simulink model "nid_cvst_ir"  (Simulink 7.6)
settings: Solver=FixedStepDiscrete  StartTime=0.0  StopTime=inf  RelTol=1e-3
libraries: vipsnks x2, nid_lib x2
settings Model: Creator=tchikama  LastModifiedBy=tchikama
settings DataIOCC: SaveOutput=off
settings OptimizationCC: SimCompilerOptimization=On
settings HardwareCC: ProdIntDivRoundTo=Zero  ProdEndianess=LittleEndian  ProdHWDeviceType=Generic->32-bit x86 compatible
settings RTWCC: ProcessScript=grt_make_rtw_hook  RTWCompilerOptimization=On
settings CodeAppCC: MaxIdLength=95

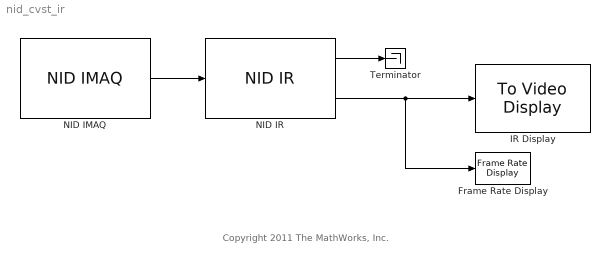
== system nid_cvst_ir ==
  note: Copyright 2011 The MathWorks, Inc.
  Frame Rate Display : vipsnks/Frame Rate Display  DialogController=vipDDGCreate  DialogControllerArgs=DataTag0  UpdateRate=10
  IR Display : vipsnks/To Video Display  DialogControllerArgs=DataTag1  inputType=Obsolete  imagePorts=One multidimensional signal  OutputDevice=On-screen video monitor  fullScreen=off  videoWindowX=880  videoWindowY=60  saveWindowSize=off  videoWindowWidth=639  videoWindowHeight=480  dataOrg=Column-major  openAtMdlStart=on  isWindowOpen=on
  NID IMAQ : nid_lib/NID IMAQ  imaq_depth=off  imaq_motion=off  imaq_image=off  view_point=off  imaq_skeleton=off  imaq_ir=on  mirror_image=off  imaq_sample_time=1/30  res_fps=VGA (640x480): 30 FPS  angle=0  angle_read=off  near_mode=off
  NID IR : nid_lib/NID IR  viewer=on
  Terminator : Terminator
  wires:
  NID IMAQ/1 -> NID IR/1
  NID IR/2 -> IR Display/1, Frame Rate Display/1
  NID IR/1 -> Terminator/1
